simulink model "Problema2_3"  (R2021b)
settings: Solver=ode4  StartTime=0.0  StopTime=20.0  FixedStep=0.01  RelTol=1e-3
values from neighbouring files (symbols this model uses):
  A = [0, 0, 0; 1, 0, -1; 0, 1, 2]    [Problema1.m]    (also in Problema1_v2.m)
  B = [0, -1; 1, 0; 0, 1]    [Problema1.m]    (also in Problema1_v2.m)
  C = [1, 0, 1]    [Problema1.m]    (also in Problema1_v2.m)
  F = F0 + g * f    [Problema1.m]    (also in Problema1_v2.m)
  G = eye(m)    [Problema1.m]    (also in Problema1_v2.m)
settings Model: Creator=Stefan  LastModifiedBy=Stefan

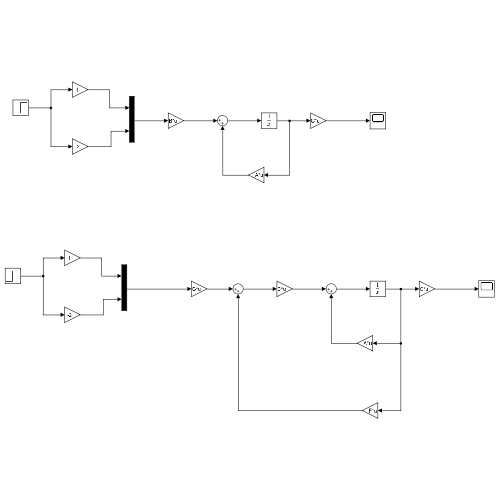
[thumbnail: Simulink's stored preview of the top-level diagram]
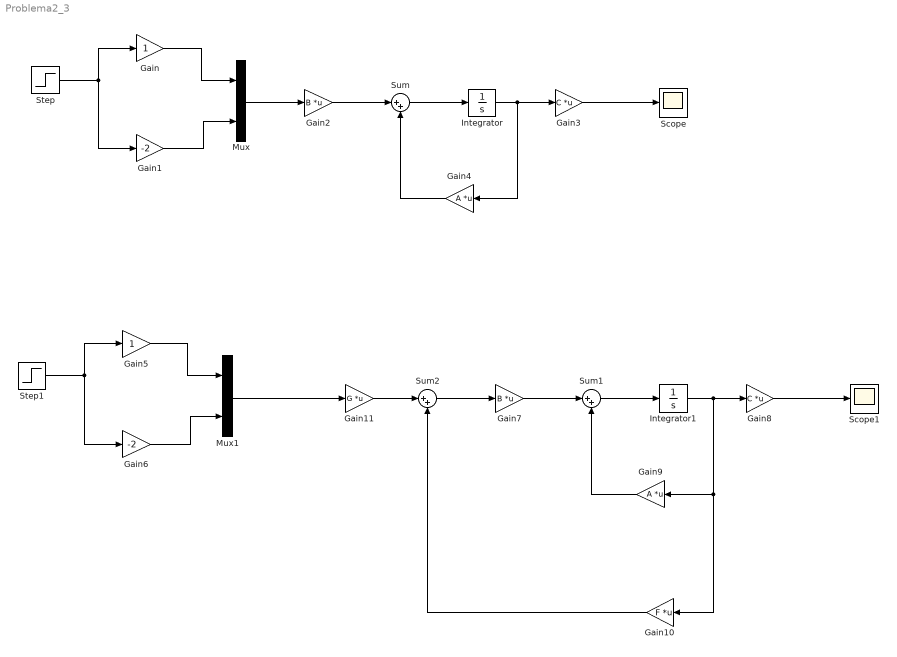
== system Problema2_3 ==
  Gain : Gain
  Gain1 : Gain  Gain=-2
  Gain10 : Gain  Gain=F  Multiplication=Matrix(K*u)
  Gain11 : Gain  Gain=G  Multiplication=Matrix(K*u)
  Gain2 : Gain  Gain=B  Multiplication=Matrix(K*u)
  Gain3 : Gain  Gain=C  Multiplication=Matrix(K*u)
  Gain4 : Gain  Gain=A  Multiplication=Matrix(K*u)
  Gain5 : Gain
  Gain6 : Gain  Gain=-2
  Gain7 : Gain  Gain=B  Multiplication=Matrix(K*u)
  Gain8 : Gain  Gain=C  Multiplication=Matrix(K*u)
  Gain9 : Gain  Gain=A  Multiplication=Matrix(K*u)
  Integrator : Integrator
  Integrator1 : Integrator
  Mux : Mux  Inputs=2
  Mux1 : Mux  Inputs=2
  Scope : Scope
  Scope1 : Scope
  Step : Step  SampleTime=0
  Step1 : Step  SampleTime=0
  Sum : Sum  Inputs=|++
  Sum1 : Sum  Inputs=|++
  Sum2 : Sum  Inputs=|++
  wires:
  Step/1 -> Gain/1, Gain1/1
  Gain1/1 -> Mux/2
  Gain/1 -> Mux/1
  Mux/1 -> Gain2/1
  Gain2/1 -> Sum/1
  Sum/1 -> Integrator/1
  Integrator/1 -> Gain4/1, Gain3/1
  Gain3/1 -> Scope/1
  Gain4/1 -> Sum/2
  Gain9/1 -> Sum1/2
  Gain5/1 -> Mux1/1
  Step1/1 -> Gain5/1, Gain6/1
  Sum1/1 -> Integrator1/1
  Integrator1/1 -> Gain10/1, Gain9/1, Gain8/1
  Gain8/1 -> Scope1/1
  Gain6/1 -> Mux1/2
  Gain7/1 -> Sum1/1
  Mux1/1 -> Gain11/1
  Gain11/1 -> Sum2/1
  Sum2/1 -> Gain7/1
  Gain10/1 -> Sum2/2
